simulink model "atraso"  (R2018a)
settings: Solver=FixedStepAuto  StartTime=0.0  StopTime=35  FixedStep=0.025  RelTol=1e-3
undefined symbols (not defined in the file): C, C1, Filtro, G
libraries: arduino_io_lib x5, simulink x1
settings Model: Creator=Mauricio  LastModifiedBy=Mauricio

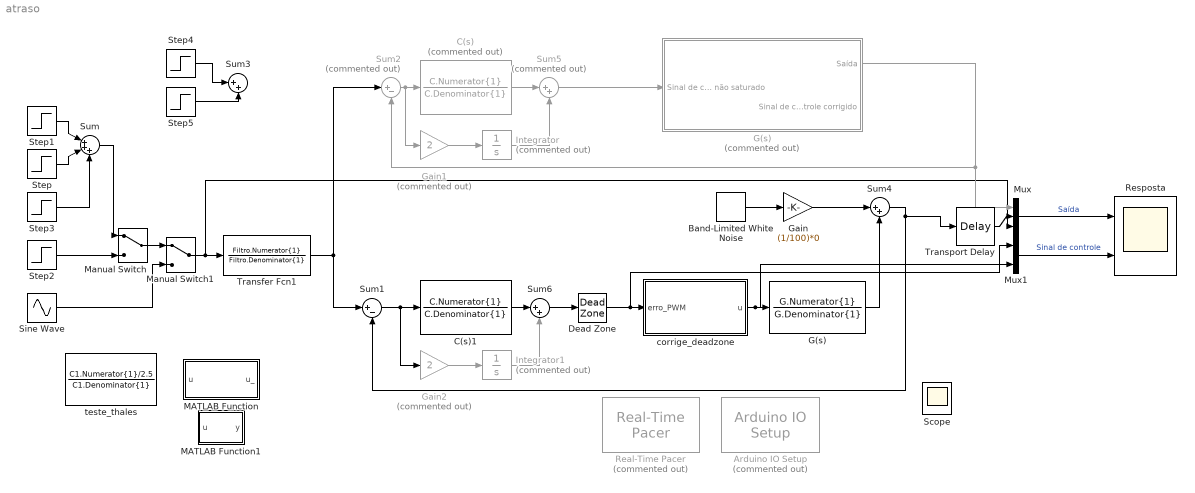
== system atraso ==
  Arduino IO Setup : arduino_io_lib/Arduino IO Setup  Priority=3  Commented=on  arduinoVar=Temporary arduino variable: Arduino1  workspaceVarName=a  comPort=COM6
  Band-Limited White Noise : simulink/Sources/Band-Limited White Noise  Cov=[0.1]  Ts=0.025  seed=[23341]
  C(s) : TransferFcn  Commented=on  Numerator=C.Numerator{1}  Denominator=C.Denominator{1}
  C(s)1 : TransferFcn  Numerator=C.Numerator{1}  Denominator=C.Denominator{1}
  Dead Zone : DeadZone  SaturateOnIntegerOverflow=on
  G(s) : TransferFcn  Numerator=G.Numerator{1}  Denominator=G.Denominator{1}
  "G(s) " : Subsystem  Commented=on
  Gain : Gain  Gain=(1/100)*0
  Gain1 : Gain  Commented=on  Gain=2
  Gain2 : Gain  Commented=on  Gain=2
  Integrator : Integrator  Commented=on
  Integrator1 : Integrator  Commented=on
  MATLAB Function : MATLAB Function  TreatAsAtomicUnit=on
  MATLAB Function1 : MATLAB Function  TreatAsAtomicUnit=on
  Manual Switch : ManualSwitch
  Manual Switch1 : ManualSwitch
  Mux : Mux  Inputs=3
  Mux1 : Mux  Inputs=2
  Real-Time Pacer : arduino_io_lib/Real-Time Pacer  Commented=on  simTimePerRealTime=1
  Resposta : Scope  NumInputPorts=2
  Scope : Scope  NumInputPorts=3
  Sine Wave : Sin  Amplitude=6  Frequency=2.5
  Step : Step  Time=15  After=3
  Step1 : Step  Time=5  After=3
  Step2 : Step  Time=0  After=0
  Step3 : Step  Time=25  After=-6
  Step4 : Step  After=-2  SampleTime=0
  Step5 : Step  Time=10  After=4  SampleTime=0
  Sum : Sum  Inputs=|+++
  Sum1 : Sum  Inputs=|+-
  Sum2 : Sum  Commented=on  Inputs=|+-
  Sum3 : Sum  Inputs=|++
  Sum4 : Sum  Inputs=|++
  Sum5 : Sum  Commented=on  Inputs=|++
  Sum6 : Sum  Inputs=|++
  Transfer Fcn1 : TransferFcn  Numerator=Filtro.Numerator{1}  Denominator=Filtro.Denominator{1}
  Transport Delay : TransportDelay  DelayTime=0
  corrige_deadzone : MATLAB Function  TreatAsAtomicUnit=on
  teste_thales : TransferFcn  Numerator=C1.Numerator{1}/2.5  Denominator=C1.Denominator{1}
  wires:
  Sum2/1 -> Gain1/1, C(s)/1
  Step1/1 -> Sum/1
  Step2/1 -> Manual Switch/2
  Step/1 -> Sum/2
  Step3/1 -> Sum/3
  Manual Switch/1 -> Manual Switch1/1
  Sine Wave/1 -> Manual Switch1/2
  Manual Switch1/1 -> Mux/3, Transfer Fcn1/1
  Step4/1 -> Sum3/1
  Step5/1 -> Sum3/2
  Sum/1 -> Manual Switch/1
  Transfer Fcn1/1 -> Sum1/1, Sum2/1
  "G(s) "/1(Saída) -> Mux/1, Sum2/2
  Mux/1 -> Resposta/1  "Saída"
  Mux1/1 -> Resposta/2  "Sinal de controle"
  Band-Limited White Noise/1 -> Gain/1
  Sum4/1 -> Sum1/2, Transport Delay/1
  Gain/1 -> Sum4/1
  C(s)/1 -> Sum5/1
  Integrator/1 -> Sum5/2
  Gain1/1 -> Integrator/1
  Sum5/1 -> "G(s) "/1(Sinal de controle não saturado)
  Sum1/1 -> Gain2/1, C(s)1/1
  Gain2/1 -> Integrator1/1
  Integrator1/1 -> Sum6/2
  C(s)1/1 -> Sum6/1
  Sum6/1 -> Dead Zone/1
  corrige_deadzone/1(u) -> G(s)/1, Mux1/2
  G(s)/1 -> Sum4/2
  Transport Delay/1 -> Mux/2
  Dead Zone/1 -> Mux1/1, corrige_deadzone/1(erro_PWM)

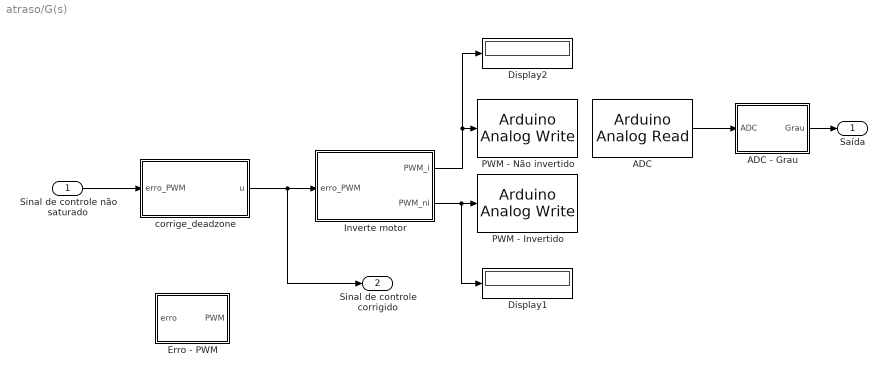
== system atraso/G(s)  ==
  Sinal de controle não saturado : Inport
  ADC : arduino_io_lib/Arduino Analog Read  arduinoVar=Temporary arduino variable: Arduino1  arduinoPin=2  T=0.025
  ADC - Grau : MATLAB Function  TreatAsAtomicUnit=on
  Display1 : Display
  Display2 : Display
  Erro - PWM : MATLAB Function  TreatAsAtomicUnit=on
  Inverte motor : MATLAB Function  TreatAsAtomicUnit=on
  PWM - Invertido : arduino_io_lib/Arduino Analog Write  arduinoVar=Temporary arduino variable: Arduino1  arduinoPin=6  T=0.025
  PWM - Não invertido : arduino_io_lib/Arduino Analog Write  arduinoVar=Temporary arduino variable: Arduino1  arduinoPin=5  T=0.025
  corrige_deadzone : MATLAB Function  TreatAsAtomicUnit=on
  Saída : Outport
  Sinal de controle corrigido : Outport  Port=2
  wires:
  ADC/1 -> ADC - Grau/1(ADC)
  Inverte motor/2(PWM_ni) -> Display1/1, PWM - Invertido/1
  Inverte motor/1(PWM_i) -> Display2/1, PWM - Não invertido/1
  ADC - Grau/1(Grau) -> Saída/1
  Sinal de controle não saturado/1 -> corrige_deadzone/1(erro_PWM)
  corrige_deadzone/1(u) -> Sinal de controle corrigido/1, Inverte motor/1(erro_PWM)

== matlab function atraso/MATLAB Function ==
  data: u input; u_ output
function u_ = dead_zone(u)
dz = 45;
if(abs(u)<=dz)
    u_=0;
else
    u_=u;
end

== matlab function atraso/G(s) /Erro - PWM ==
  data: erro input; PWM output
function PWM = fcn(erro)

if(erro < pi/180 && erro >=0)
    PWM = 0;
elseif(erro > -pi/180 && erro < 0)
    PWM = 0;
else
    PWM = 150.7783671396903180968372495108*erro + 57.368421052631578947368421052632;
end

== matlab function atraso/corrige_deadzone ==
  data: u output; erro_PWM input
function u  = fcn(erro_PWM)
dead_zoneN = -35;
dead_zoneP = 35;

%Corrigindo a zona morta
if(erro_PWM < 0)
    u = erro_PWM + dead_zoneN;
% DESLIGADO
else
    u = erro_PWM + dead_zoneP;
end
% function u  = fcn(erro_PWM)
% dead_zone = 40;
% erro_adm = 0;
% % erro_permissivel = 0.5;
% % 
% % % Confere se a saída está dentro de um erro aceitável, já que não tem
% % % integrador no controlador
% 
% %Corrigindo a zona morta
% if(erro_adm < abs(erro_PWM) && abs(erro_PWM) < dead_zone)
%     u = erro_PWM + dead_zone;
% % DESLIGADO
% elseif(abs(erro_PWM) <= erro_adm)
%     u=0;
% else
%     u=erro_PWM;
% end

== matlab function atraso/G(s) /ADC - Grau ==
  data: ADC input; Grau output
function Grau = fcn(ADC)
Grau = -0.17413322126497163269594452616096*ADC + 136.2690584156335364572389157386;

== matlab function atraso/G(s) /Inverte motor ==
  data: PWM_i output; PWM_ni output; erro_PWM input
function [PWM_i, PWM_ni] = fcn(erro_PWM)

%REVERSO
if(erro_PWM>0)
    PWM_i = erro_PWM;
    PWM_ni = 0;
%FRENTE
elseif(erro_PWM<0)
    PWM_ni = abs(erro_PWM);
    PWM_i = 0;
%DESLIGADO
else
    PWM_ni = 0;
    PWM_i = 0;
end

== matlab function atraso/G(s) /corrige_deadzone ==
  data: u output; erro_PWM input
function u  = fcn(erro_PWM)
dead_zoneN = -25;
dead_zoneP = 25;

%Corrigindo a zona morta
if(erro_PWM < 0)
    u = erro_PWM + dead_zoneN;
% DESLIGADO
else
    u = erro_PWM + dead_zoneP;
end
% function u  = fcn(erro_PWM)
% dead_zone = 40;
% erro_adm = 0;
% % erro_permissivel = 0.5;
% % 
% % % Confere se a saída está dentro de um erro aceitável, já que não tem
% % % integrador no controlador
% 
% %Corrigindo a zona morta
% if(erro_adm < abs(erro_PWM) && abs(erro_PWM) < dead_zone)
%     u = erro_PWM + dead_zone;
% % DESLIGADO
% elseif(abs(erro_PWM) <= erro_adm)
%     u=0;
% else
%     u=erro_PWM;
% end

== matlab function atraso/MATLAB Function1 ==
  data: u input; y output
function y = fcn(u)
dz = 35;
if abs(u)<=dz
    y = 0;
else
    y = u;
end
